simulink model "example_quadcopter_agressive"  (R2016a)
settings: Solver=VariableStepAuto  StartTime=0.0  StopTime=15  RelTol=1e-3
settings Model: Creator=Daniel  LastModifiedBy=mgreiff
settings DataIOCC: LimitDataPoints=on
settings DebuggingCC: AllowSymbolicDim=off
settings ModelReferenceCC: PropagateSignalLabelsOutOfModel=off
settings GRTTargetCC: GeneratePreprocessorConditionals=Use local settings

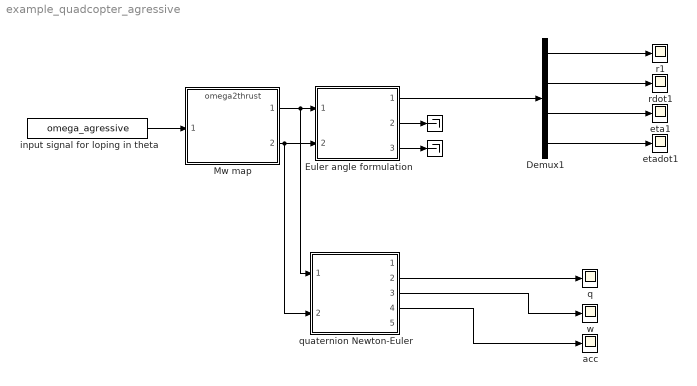
== system example_quadcopter_agressive ==
  " " : Terminator
  "  " : Terminator
  Demux1 : Demux  Outputs=[3,3,3,3]
  Euler angle formulation : ModelReference  ModelNameDialog=quadcopter_model_c_Euler.mdl  SimulationMode=Normal  ModelReferenceVersion=1.167
  Mw map : ModelReference  ModelNameDialog=omega2thrust.mdl  SimulationMode=Normal  ModelReferenceVersion=1.3
  acc : Scope
  eta1 : Scope
  etadot1 : Scope
  input signal for loping in theta : FromFile  FileName=omega_agressive  ExtrapolationBeforeFirstDataPoint=Hold first value
  q : Scope
  quaternion Newton-Euler : ModelReference  ModelNameDialog=quadcopter_model_c_NewtonEuler.mdl  SimulationMode=Normal  ModelReferenceVersion=1.325
  r1 : Scope
  rdot1 : Scope
  w : Scope
  wires:
  input signal for loping in theta/1 -> Mw map/1
  Euler angle formulation/2 -> " "/1
  Euler angle formulation/3 -> "  "/1
  Euler angle formulation/1 -> Demux1/1
  Demux1/3 -> eta1/1
  Demux1/2 -> rdot1/1
  Demux1/1 -> r1/1
  Demux1/4 -> etadot1/1
  Mw map/2 -> quaternion Newton-Euler/2, Euler angle formulation/2
  Mw map/1 -> quaternion Newton-Euler/1, Euler angle formulation/1
  quaternion Newton-Euler/4 -> acc/1
  quaternion Newton-Euler/2 -> q/1
  quaternion Newton-Euler/3 -> w/1
